simulink model "freqOscillations"  (R2014a)
settings: Solver=ode45  StartTime=0.0  StopTime=10.0  RelTol=1e-3
settings Model: Creator=Grid  LastModifiedBy=Grid

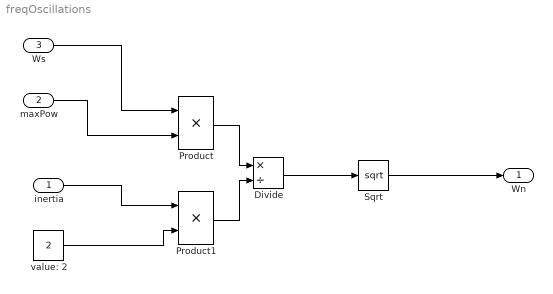
== system freqOscillations ==
  inertia : Inport
  maxPow : Inport  Port=2
  Ws : Inport  Port=3
  Divide : Product  Inputs=*/
  Product : Product
  Product1 : Product
  Sqrt : Sqrt  SaturateOnIntegerOverflow=on
  "value: 2 " : Constant  Value=2
  Wn : Outport  RequirementInfo={'linktype_rmi_matlab' 'Diesel' '@736250.1' 'true' 'freqOscillations' '' } %GIDa_0f6f51fa_a55b_4ce9_89e4_107fbcc432ac
  wires:
  Ws/1 -> Product/1
  maxPow/1 -> Product/2
  inertia/1 -> Product1/1
  "value: 2 "/1 -> Product1/2
  Product/1 -> Divide/1
  Product1/1 -> Divide/2
  Divide/1 -> Sqrt/1
  Sqrt/1 -> Wn/1
